simulink model "dynamic_model_euler_copy_to_compare"  (R2021b)
settings: Solver=FixedStepAuto  StartTime=0.0  StopTime=simTime  FixedStep=sim_dt  RelTol=1e-3
undefined symbols (not defined in the file): Angle, Axis, d, g, J_platf, m_mass, m_platf, p, q0, roff, sim_dt, tau, time_1, time_2, u0, umax, w0
libraries: sharedtransform x2, simulink x1, robotcorelib x1, dspindex x1, matrix_library x1
settings Model: Creator=piszy  LastModifiedBy=krzysztof
settings SolverCC: ZeroCrossControl=DisableAll  AlgebraicLoopSolver=TrustRegion
settings DataIOCC: SaveOutput=off  SaveTime=off
settings OptimizationCC: BlockReduction=off  DefaultParameterBehavior=Inlined  BufferReuse=off
settings ModelReferenceCC: ModelReferenceNumInstancesAllowed=Single
settings SFSimCC: CustomCodeUndefinedFunction=UseInterfaceOnly
settings GRTTargetCC: CombineOutputUpdateFcns=off  MatFileLogging=off

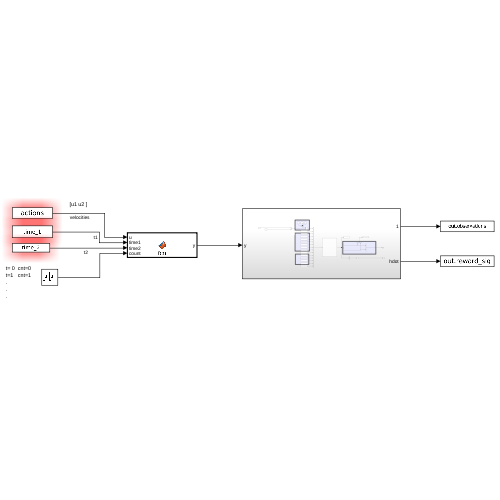
[thumbnail: Simulink's stored preview of the top-level diagram]
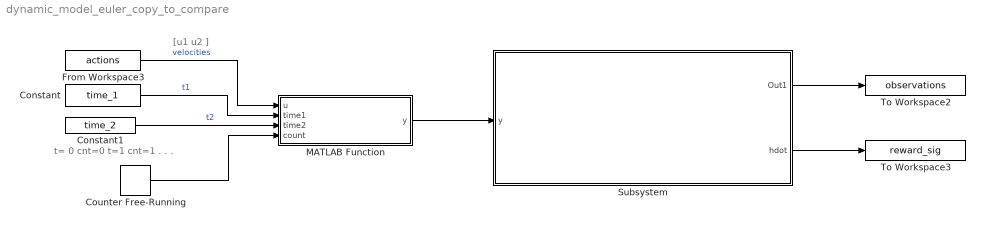
== system dynamic_model_euler_copy_to_compare ==
  note: t= 0  cnt=0
      | t=1   cnt=1
      | .
      | .
      | .
  note: [u1 u2 ]
  Constant : Constant  Value=time_1
  Constant1 : Constant  Value=time_2
  Counter Free-Running : simulink/Sources/Counter Free-Running  NumBits=16  tsamp=-1
  From Workspace3 : FromWorkspace  VariableName=actions
  MATLAB Function : MATLAB Function  TreatAsAtomicUnit=on
  Subsystem : Subsystem
  To Workspace2 : ToWorkspace  VariableName=observations  SampleTime=-1
  To Workspace3 : ToWorkspace  VariableName=reward_sig  SampleTime=-1
  wires:
  Subsystem/1(Out1) -> To Workspace2/1
  Subsystem/2(hdot) -> To Workspace3/1
  From Workspace3/1 -> MATLAB Function/1(u)  "velocities"
  MATLAB Function/1(y) -> Subsystem/1(y)
  Constant/1 -> MATLAB Function/2(time1)  "t1"
  Constant1/1 -> MATLAB Function/3(time2)  "t2"
  Counter Free-Running/1 -> MATLAB Function/4(count)

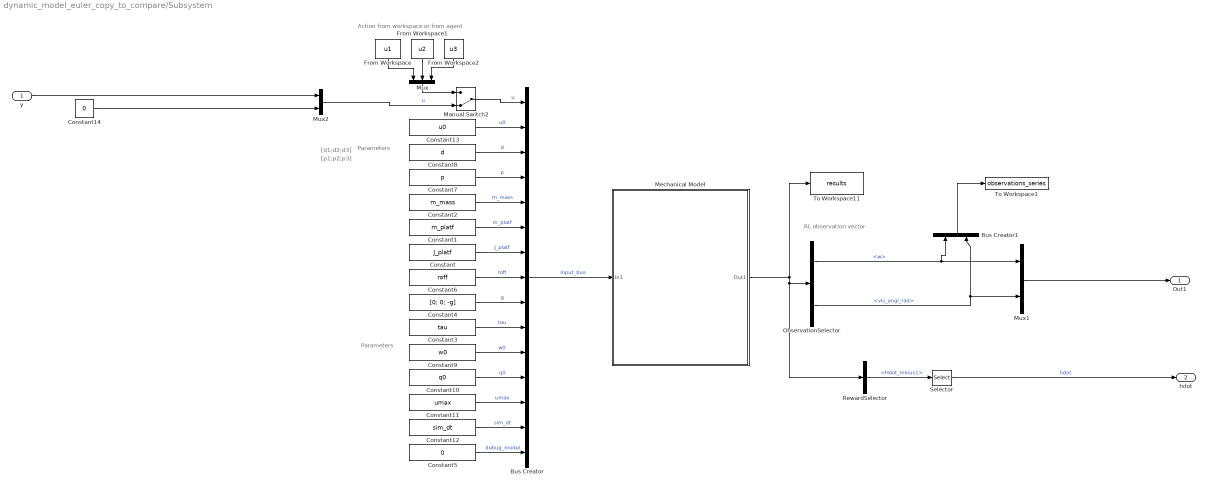
== system dynamic_model_euler_copy_to_compare/Subsystem ==
  note: Parameters
  note: Action from workspace or from agent
  note: RL observation vector
  note: [p1;p2;p3]
  note: [d1;d2;d3]
  note: Parameters
  y : Inport
  Bus Creator : BusCreator  Inputs=15
  Bus Creator1 : BusCreator  Inputs=2
  Constant : Constant  Value=J_platf
  Constant1 : Constant  Value=m_platf
  Constant10 : Constant  Value=q0
  Constant11 : Constant  Value=umax
  Constant12 : Constant  Value=sim_dt
  Constant13 : Constant  Value=u0
  Constant14 : Constant  Value=0
  Constant2 : Constant  Value=m_mass
  Constant3 : Constant  Value=tau
  Constant4 : Constant  Value=[0; 0; -g]
  Constant5 : Constant  Value=0
  Constant6 : Constant  Value=roff
  Constant7 : Constant  Value=p
  Constant8 : Constant  Value=d
  Constant9 : Constant  Value=w0
  From Workspace : FromWorkspace  VariableName=u1
  From Workspace1 : FromWorkspace  VariableName=u2
  From Workspace2 : FromWorkspace  VariableName=u3
  Manual Switch2 : ManualSwitch  CurrentSetting=0
  Mechanical Model : Subsystem
  Mux : Mux  Inputs=3
  Mux1 : Mux  Inputs=2
  Mux2 : Mux  Inputs=2
  ObservationSelector : BusSelector  OutputSignals=w,vis_angl_rad
  RewardSelector : BusSelector  OutputSignals=Hdot_minus1
  Selector : Selector  InputPortWidth=3  IndexOptions=Index vector (dialog)  Indices=[3]  OutputSizes=1
  To Workspace1 : ToWorkspace  VariableName=observations_series  SaveFormat=Timeseries  SampleTime=-1
      settings: Save2DSignal=2-D array (concatenate along first dimension)
  To Workspace11 : ToWorkspace  VariableName=results  SaveFormat=Timeseries  SampleTime=-1
      settings: Save2DSignal=2-D array (concatenate along first dimension)
  Out1 : Outport
  hdot : Outport  Port=2
  wires:
  Constant10/1 -> Bus Creator/12  "q0"
  Constant2/1 -> Bus Creator/5  "m_mass"
  Constant14/1 -> Mux2/2
  Constant11/1 -> Bus Creator/13  "umax"
  Constant13/1 -> Bus Creator/2  "u0"
  Bus Creator1/1 -> To Workspace1/1
  Constant9/1 -> Bus Creator/11  "w0"
  Constant1/1 -> Bus Creator/6  "m_platf"
  Constant7/1 -> Bus Creator/4  "p"
  Constant3/1 -> Bus Creator/10  "tau"
  Constant4/1 -> Bus Creator/9  "g"
  y/1 -> Mux2/1
  Constant6/1 -> Bus Creator/8  "roff"
  ObservationSelector/1 -> Bus Creator1/1, Mux1/1  "<w>"
  Constant12/1 -> Bus Creator/14  "sim_dt"
  Mux1/1 -> Out1/1
  Mechanical Model/1(Out1) -> To Workspace11/1, ObservationSelector/1, RewardSelector/1
  Selector/1 -> hdot/1  "hdot"
  Constant5/1 -> Bus Creator/15  "debug_model"
  Constant/1 -> Bus Creator/7  "J_platf"
  RewardSelector/1 -> Selector/1  "<Hdot_minus1>"
  Constant8/1 -> Bus Creator/3  "d"
  ObservationSelector/2 -> Bus Creator1/2, Mux1/2  "<vis_angl_rad>"
  From Workspace2/1 -> Mux/3
  From Workspace1/1 -> Mux/2
  From Workspace/1 -> Mux/1
  Bus Creator/1 -> Mechanical Model/1(In1)  "input_bus"
  Mux2/1 -> Manual Switch2/2  "u"
  Mux/1 -> Manual Switch2/1
  Manual Switch2/1 -> Bus Creator/1  "u"

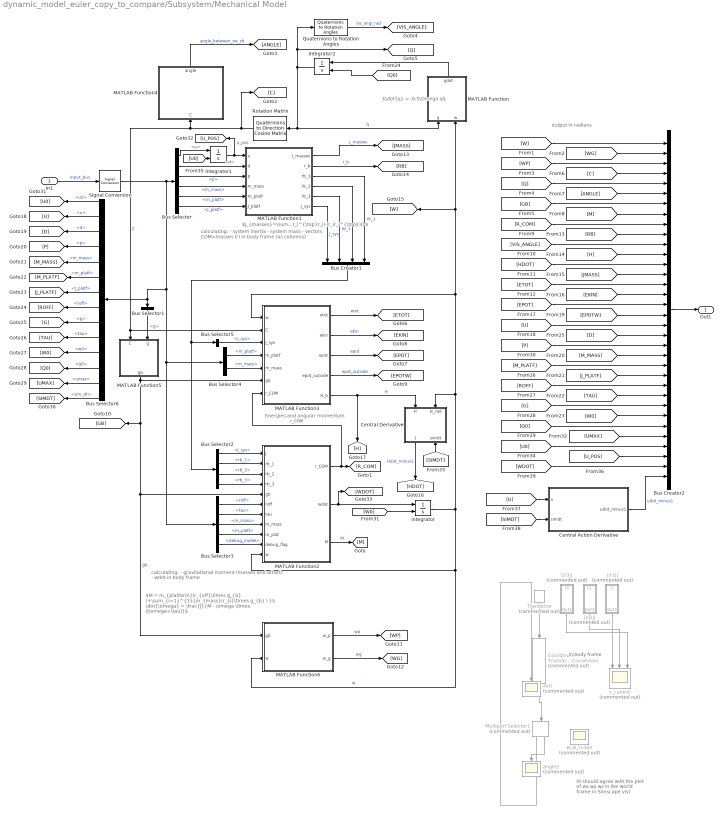
== system dynamic_model_euler_copy_to_compare/Subsystem/Mechanical Model ==
  note: $J_{masses}=\sum_{i=1}^{3}{m_{i}(I(r_i^{\top}r_i)-(r_ir_i^{\top}))}$
  note: $\dot{q} = -0.5\Omega q$
  note: $M = m_{platform}(r_{off}\times g_{b} )+\sum_{i=1}^{3}{m_{mass}(r_{i}\times g_{b} ) }\\ \dot{\omega} = \frac{J}{M - \omega \times (J\omega+\tau)}$
  note: (it should agree with the plot of wx wy wz in the world frame in Simscape vis)
  note: calculating:
      | - system inertia
      | - system mass
      | - vectors COM>masses (r) in body frame
      | (as columns)
  note: calculating:
      | - gravitational moment (masses and offset)
      | - wdot
      | in body frame
  note: in body frame
  note: Energies and angular momentum
  note: output in radians
  In1 : Inport
  Bus Creator1 : BusCreator  Inputs=4
  Bus Creator2 : BusCreator  Inputs=34
  Bus Selector : BusSelector  OutputSignals=u,d,p,m_mass,m_platf,J_platf
  Bus Selector1 : BusSelector  OutputSignals=g
  Bus Selector2 : BusSelector  OutputSignals=J_sys,rb_1,rb_2,rb_3
  Bus Selector3 : BusSelector  OutputSignals=roff,tau,m_mass,m_platf,debug_model
  Bus Selector4 : BusSelector  OutputSignals=m_platf,m_mass
  Bus Selector5 : BusSelector  OutputSignals=J_sys
  Bus Selector6 : BusSelector  OutputSignals=u0,u,d,p,m_mass,m_platf,J_platf,roff,g,tau,w0,q0,umax,sim_dt
  Central Action Derivative : Subsystem
  Central Derivative : Subsystem
      settings: PortSchema="{\"entries\":[{\"content\":{\"sides\":[{\"content\":{\"connectorIds\":[\"In1\",\"In2\"]},\"type\":\"ConnectorPlacement.EquallySpacedRectSide\",\"uuid\":\"1383cf58-ed2e-4d76-b2bd-bc812874c5c5\"},{\"content\":{\"connectorIds\":[\"Out1\",\"In3\"],\"side\":\"RIGHT\"},\"type\":\"ConnectorPlacement.EquallySpacedRectSide\",\"uuid\":\"b1333be6-c310-4c35-a541-4e98fbac6c75\"},{\"content\":{\"connectorIds\":[],\"side\":\"TOP\"},\"type\":\"ConnectorPlacement.EquallySpacedRectSide\",\"uuid\":\"9de10ece-9fa2-48e9-be23-db895089292f\"}]},\"type\":\"ConnectorPlacement.EquallySpacedConnector\",\"uuid\":\"8dd4b87f-23e7-464d-a0c4-c49a8f880c8a\"}],\"packageUris\":[\"http://schema.mathworks.com/mf0/Connector/R2020b\"],\"version\":\"1.0\"}"
  Coordinate Transformation Conversion : robotcorelib/Coordinate Transformation Conversion  Commented=on  InputRepresentation=Rotation Matrix  InputEulerSequence=ZYX  ShowTrVecInputPort=on  OutputRepresentation=Axis-Angle  OutputEulerSequence=ZYX  ShowTrVecOutputPort=on  SimulateUsing=Interpreted execution
      settings: SourceProductBaseCode=NV,RO,RR,UV
  Integrator : Integrator  InitialConditionSource=external
  Integrator1 : Integrator  InitialConditionSource=external
  Integrator2 : Integrator  InitialConditionSource=external
  MATLAB Function : MATLAB Function  TreatAsAtomicUnit=on
  MATLAB Function1 : MATLAB Function  TreatAsAtomicUnit=on
  MATLAB Function2 : MATLAB Function  TreatAsAtomicUnit=on
  MATLAB Function3 : MATLAB Function  TreatAsAtomicUnit=on
  MATLAB Function4 : MATLAB Function  TreatAsAtomicUnit=on
  MATLAB Function5 : MATLAB Function  TreatAsAtomicUnit=on
  MATLAB Function6 : MATLAB Function  TreatAsAtomicUnit=on
  Multiport Selector1 : dspindex/Multiport Selector  Commented=on  rowsOrCols=Rows  idxCellArray={1:3,4}  idxErrMode=Clip Index
  Quaternions to Rotation Angles : sharedtransform/Quaternions to Rotation Angles  rotationOrder=XYZ  aMode=aMode
      settings: SourceProductBaseCode=AE,PW,DR,MT,UV,VE
  Rotation Matrix : sharedtransform/Quaternions to  Direction Cosine Matrix  aMode=aMode
      settings: SourceProductBaseCode=AE,PW,DR,MT,UV,VE
  Signal Conversion : SignalConversion  OverrideOpt=on
  Transpose : matrix_library/Transpose  Commented=on
      settings: SourceProductBaseCode=SL
  angle2 : Scope  Commented=on
  axis : Scope  Commented=on
  r_control : Scope  Commented=on  NumInputPorts=3
  w_w_scope : Scope  Commented=on
  ||r1|| : Subsystem  Commented=on
  ||r2|| : Subsystem  Commented=on
  ||r3|| : Subsystem  Commented=on
  Out1 : Outport
  wires:
  Integrator2/1 -> MATLAB Function/1(q), Rotation Matrix/1, [Q], Quaternions to Rotation Angles/1  "q"
  MATLAB Function/1(qdot) -> Integrator2/1
  Transpose/1 -> Coordinate Transformation Conversion/1
  Coordinate Transformation Conversion/1 -> Multiport Selector1/1
  Multiport Selector1/2 -> angle2/1
  Multiport Selector1/1 -> axis/1
  ||r3||/1(Out1) -> r_control/3
  ||r1||/1(Out1) -> r_control/1
  ||r2||/1(Out1) -> r_control/2
  In1/1 -> Signal Conversion/1  "input_bus"
  Bus Selector/2 -> MATLAB Function1/2(d)  "<d>"
  Bus Selector/3 -> MATLAB Function1/3(p)  "<p>"
  Bus Selector/4 -> MATLAB Function1/4(m_mass)  "<m_mass>"
  Bus Selector/5 -> MATLAB Function1/5(m_platf)  "<m_platf>"
  Bus Selector1/1 -> MATLAB Function5/2(g)  "<g>"
  MATLAB Function2/2(wdot) -> Integrator/1, [WDOT]
  Integrator/1 -> MATLAB Function6/2(w), MATLAB Function2/11(w), MATLAB Function3/1(w), [W], MATLAB Function/2(w), Central Derivative/2(w_rad)  "w"
  MATLAB Function1/3(rb_1) -> Bus Creator1/4  "rb_1"
  MATLAB Function5/1(gb) -> MATLAB Function6/1(gb), MATLAB Function2/5(gb), [GB], MATLAB Function3/6(gb)  "gb"
  MATLAB Function1/4(rb_2) -> Bus Creator1/3  "rb_2"
  MATLAB Function1/5(rb_3) -> Bus Creator1/2  "rb_3"
  MATLAB Function1/6(J_sys) -> Bus Creator1/1  "J_sys"
  Bus Selector3/1 -> MATLAB Function2/6(roff)  "<roff>"
  Bus Selector3/2 -> MATLAB Function2/7(tau)  "<tau>"
  Bus Selector3/3 -> MATLAB Function2/8(m_mass)  "<m_mass>"
  Bus Selector3/4 -> MATLAB Function2/9(m_plat)  "<m_platf>"
  Bus Creator1/1 -> Bus Selector5/1, Bus Selector2/1
  MATLAB Function2/3(M) -> [M]  "M"
  MATLAB Function3/2(ekin) -> [EKIN]  "ekin"
  MATLAB Function3/3(epot) -> [EPOT]  "epot"
  MATLAB Function3/1(etot) -> [ETOT]  "etot"
  MATLAB Function6/1(w_p) -> [WP]  "wp"
  MATLAB Function6/2(w_g) -> [WG]  "wg"
  MATLAB Function1/1(J_masses) -> [JMASS]  "J_masses"
  Bus Selector/6 -> MATLAB Function1/6(J_platf)  "<J_platf>"
  Bus Selector3/5 -> MATLAB Function2/10(debug_flag)  "<debug_model>"
  Bus Selector4/2 -> MATLAB Function3/5(m_mass)  "<m_mass>"
  Bus Selector4/1 -> MATLAB Function3/4(m_platf)  "<m_platf>"
  MATLAB Function2/1(r_COM) -> [R_COM], MATLAB Function3/7(r_COM)  "r_COM"
  Bus Selector2/1 -> MATLAB Function2/1(J)  "<J_sys>"
  Bus Selector2/3 -> MATLAB Function2/3(rb_2)  "<rb_2>"
  Bus Selector2/2 -> MATLAB Function2/2(rb_1)  "<rb_1>"
  Bus Selector2/4 -> MATLAB Function2/4(rb_3)  "<rb_3>"
  Bus Selector5/1 -> MATLAB Function3/3(J_sys)  "<J_sys>"
  MATLAB Function3/4(epot_outside) -> [EPOTW]  "epot_outside"
  Rotation Matrix/1 -> [C], MATLAB Function3/2(C), MATLAB Function5/1(C), MATLAB Function4/1(C)  "C"
  Bus Creator2/1 -> Out1/1
  MATLAB Function1/2(r_b) -> [RB]  "r_b"
  MATLAB Function4/1(angle) -> [ANGLE]  "angle_between_zw_zb"
  Quaternions to Rotation Angles/1 -> [VIS_ANGLE]  "vis_angl_rad"
  [W] -> Bus Creator2/1
  [WG] -> Bus Creator2/2
  [C] -> Bus Creator2/4
  [WP] -> Bus Creator2/3
  [JMASS] -> Bus Creator2/14
  [HDOT] -> Bus Creator2/13
  [H] -> Bus Creator2/12
  [VIS_ANGLE] -> Bus Creator2/11
  [R_COM] -> Bus Creator2/9
  [ETOT] -> Bus Creator2/15
  [EPOT] -> Bus Creator2/17
  [EPOTW] -> Bus Creator2/18
  [Q] -> Bus Creator2/5
  [GB] -> Bus Creator2/7
  [ANGLE] -> Bus Creator2/6
  [M] -> Bus Creator2/8
  [RB] -> Bus Creator2/10
  [EKIN] -> Bus Creator2/16
  [U] -> Bus Creator2/19
  Bus Selector6/7 -> [J_PLATF]  "<J_platf>"
  Bus Selector6/8 -> [ROFF]  "<roff>"
  Bus Selector6/9 -> [G]  "<g>"
  Bus Selector6/10 -> [TAU]  "<tau>"
  Bus Selector6/11 -> [W0]  "<w0>"
  Bus Selector6/12 -> [Q0]  "<q0>"
  Bus Selector6/6 -> [M_PLATF]  "<m_platf>"
  Bus Selector6/5 -> [M_MASS]  "<m_mass>"
  Bus Selector6/4 -> [P]  "<p>"
  Bus Selector6/3 -> [D]  "<d>"
  Bus Selector6/2 -> [U]  "<u>"
  [D] -> Bus Creator2/20
  [TAU] -> Bus Creator2/26
  [M_MASS] -> Bus Creator2/22
  [W0] -> Bus Creator2/28
  [J_PLATF] -> Bus Creator2/24
  [P] -> Bus Creator2/21
  [M_PLATF] -> Bus Creator2/23
  [ROFF] -> Bus Creator2/25
  [G] -> Bus Creator2/27
  [Q0] -> Bus Creator2/29
  [Q0] -> Integrator2/2
  [W0] -> Integrator/2
  MATLAB Function3/5(H_b) -> Central Derivative/1(H), [H]  "H"
  Central Derivative/1(Hdot_minus1) -> [HDOT]  "Hdot_minus1"
  Bus Selector6/13 -> [UMAX]  "<umax>"
  [UMAX] -> Bus Creator2/30
  Bus Selector6/14 -> [SIMDT]  "<sim_dt>"
  [SIMDT] -> Central Derivative/3(simdt)
  Signal Conversion/1 -> Bus Selector3/1, Bus Selector4/1, Bus Selector1/1, Bus Selector6/1, Bus Selector/1
  Bus Selector6/1 -> [U0]  "<u0>"
  [U0] -> Bus Creator2/31
  Bus Selector/1 -> Integrator1/1  "<u>"
  [U0] -> Integrator1/2
  Integrator1/1 -> [U_POS], MATLAB Function1/1(u)  "u_pos"
  [U_POS] -> Bus Creator2/32
  [U] -> Central Action Derivative/2(u)
  [SIMDT] -> Central Action Derivative/1(simdt)
  Central Action Derivative/1(udot_minus1) -> Bus Creator2/34  "udot_minus1"
  [WDOT] -> Bus Creator2/33

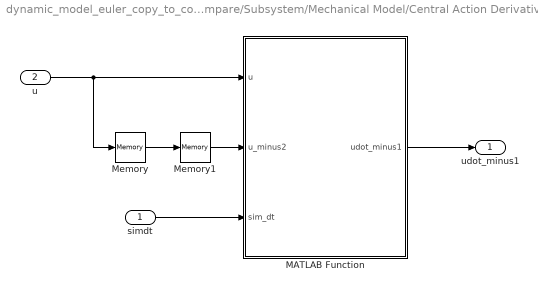
== system dynamic_model_euler_copy_to_compare/Subsystem/Mechanical Model/Central Action Derivative ==
  simdt : Inport
  u : Inport  Port=2
  MATLAB Function : MATLAB Function  TreatAsAtomicUnit=on
  Memory : Memory
  Memory1 : Memory
  udot_minus1 : Outport
  wires:
  u/1 -> Memory/1, MATLAB Function/1(u)
  simdt/1 -> MATLAB Function/3(sim_dt)
  Memory/1 -> Memory1/1
  MATLAB Function/1(udot_minus1) -> udot_minus1/1
  Memory1/1 -> MATLAB Function/2(u_minus2)

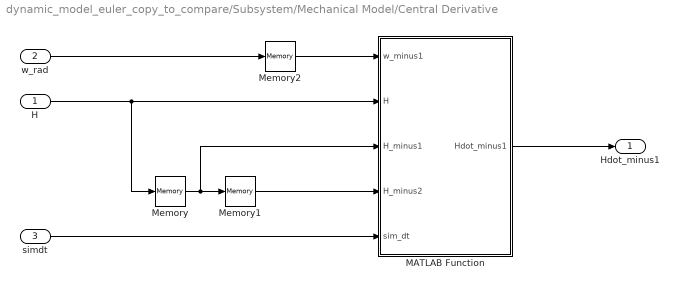
== system dynamic_model_euler_copy_to_compare/Subsystem/Mechanical Model/Central Derivative ==
  H : Inport
  w_rad : Inport  Port=2
  simdt : Inport  Port=3
  MATLAB Function : MATLAB Function  TreatAsAtomicUnit=on
  Memory : Memory
  Memory1 : Memory
  Memory2 : Memory
  Hdot_minus1 : Outport
  wires:
  Memory1/1 -> MATLAB Function/4(H_minus2)
  H/1 -> MATLAB Function/2(H), Memory/1
  Memory2/1 -> MATLAB Function/1(w_minus1)
  simdt/1 -> MATLAB Function/5(sim_dt)
  Memory/1 -> MATLAB Function/3(H_minus1), Memory1/1
  MATLAB Function/1(Hdot_minus1) -> Hdot_minus1/1
  w_rad/1 -> Memory2/1

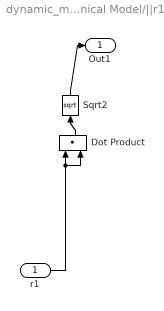
== system dynamic_model_euler_copy_to_compare/Subsystem/Mechanical Model/||r1|| ==
  r1 : Inport
  Dot Product : DotProduct  RndMeth=Nearest  InputSameDT=on  OutDataTypeStr=Inherit: Inherit via internal rule
  Sqrt2 : Sqrt  SaturateOnIntegerOverflow=on
  Out1 : Outport
  wires:
  Dot Product/1 -> Sqrt2/1
  r1/1 -> Dot Product/2, Dot Product/1
  Sqrt2/1 -> Out1/1

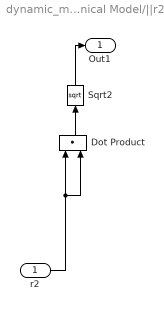
== system dynamic_model_euler_copy_to_compare/Subsystem/Mechanical Model/||r2|| ==
  r2 : Inport
  Dot Product : DotProduct  RndMeth=Nearest  InputSameDT=on  OutDataTypeStr=Inherit: Inherit via internal rule
  Sqrt2 : Sqrt  SaturateOnIntegerOverflow=on
  Out1 : Outport
  wires:
  Dot Product/1 -> Sqrt2/1
  r2/1 -> Dot Product/1, Dot Product/2
  Sqrt2/1 -> Out1/1

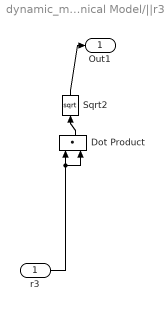
== system dynamic_model_euler_copy_to_compare/Subsystem/Mechanical Model/||r3|| ==
  r3 : Inport
  Dot Product : DotProduct  RndMeth=Nearest  InputSameDT=on  OutDataTypeStr=Inherit: Inherit via internal rule
  Sqrt2 : Sqrt  SaturateOnIntegerOverflow=on
  Out1 : Outport
  wires:
  Dot Product/1 -> Sqrt2/1
  r3/1 -> Dot Product/2, Dot Product/1
  Sqrt2/1 -> Out1/1

== matlab function dynamic_model_euler_copy_to_compare/Subsystem/Mechanical Model/Central Derivative/MATLAB Function ==
  data: w_minus1 input; H input; H_minus1 input; Hdot_minus1 output; H_minus2 input; sim_dt input
function Hdot_minus1 = fcn(w_minus1,H,H_minus1,H_minus2, sim_dt)
   H_in_body_dot_minus1 = (H - H_minus2)/2/sim_dt;
   Hdot_minus1 = H_in_body_dot_minus1 + cross(w_minus1,H_minus1);

== matlab function dynamic_model_euler_copy_to_compare/Subsystem/Mechanical Model/Central Action Derivative/MATLAB Function ==
  data: u input; u_minus2 input; udot_minus1 output; sim_dt input
function udot_minus1 = fcn(u,u_minus2, sim_dt)
   udot_minus1 = (u - u_minus2)/2/sim_dt;

== matlab function dynamic_model_euler_copy_to_compare/MATLAB Function ==
  data: u input; y output; time1 input; time2 input; count input
function y = fcn(u,time1, time2, count)
    action1 = u(1); action2 = u(2);
    y = zeros(2,1);

    if count<=time1, y(1) = action1;
    else, y(1) = 0;end

    if count<=time2, y(2) = action2;
    else, y(2) = 0;end

== matlab function dynamic_model_euler_copy_to_compare/Subsystem/Mechanical Model/MATLAB Function5 ==
  data: C input; gb output; g input
function gb = gbodyframe(C,g)
gb = C*g;

== matlab function dynamic_model_euler_copy_to_compare/Subsystem/Mechanical Model/MATLAB Function3 ==
  data: w input; C input; J_sys input; m_platf input; m_mass input; gb input; etot output; ekin output; epot output; epot_outside output; H_b output; r_COM input
function [etot,ekin,epot,epot_outside, H_b] = fcn(w,C,J_sys, m_platf,m_mass,gb,r_COM)
% J_sys = concat_in(:,1:3);
% rb1 = concat_in(:,6);
% rb2 = concat_in(:,5);
% rb3 = concat_in(:,4);

% disp(r_COM)

ekin = 0.5*(w)'*J_sys*(w);

epot = (3*m_mass + m_platf) * gb(3) * vecnorm(r_COM);
%epot = m_platf*gb(3)*vecnorm(r_COM);

r_COM_w = C'*r_COM;
epot_outside = (3*m_mass + m_platf) * vecnorm(gb) * r_COM_w(3);

etot = epot+ekin;
%hmag = vecnorm(J*w);

% H_b = [J_sys(1,1)*w(1)-J_sys(1,2)*w(2)-J_sys(1,3)*w(3); 
%     -J_sys(2,1)*w(1)+J_sys(2,2)*w(2)-J_sys(2,3)*w(3); 
%     -J_sys(3,1)*w(1)-J_sys(3,2)*w(2)+J_sys(3,3)*w(3); 
%     ];

H_b = J_sys * w;

== matlab function dynamic_model_euler_copy_to_compare/Subsystem/Mechanical Model/MATLAB Function ==
  data: q input; w input; qdot output
function qdot = derq(q,w)

w_x = w(1); w_y = w(2); w_z = w(3);

% omega = [ 0     w_z   -w_y    w_x;... 
%           -w_z   0       w_x    w_y;... 
%           w_y   -w_x    0       w_z;... 
%           -w_x   -w_y    -w_z     0];

omega = [ 0      w_x   w_y    w_z;... 
          -w_x   0    -w_z    w_y;... 
          -w_y   w_z    0    -w_x;... 
          -w_z  -w_y   w_x     0];

qdot = -0.5*omega*q;

== matlab function dynamic_model_euler_copy_to_compare/Subsystem/Mechanical Model/MATLAB Function2 ==
  data: r_COM output; J input; rb_1 input; rb_2 input; rb_3 input; gb input; roff input; tau input; m_mass input; m_plat input; debug_flag input; w input; wdot output; M output
function [r_COM, wdot, M] = fcn(J, rb_1, rb_2, rb_3, gb, roff, tau, m_mass, m_plat, debug_flag,w)

% concatenated along columns
% J = concat_in(:,1:3);
% rb_1 = concat_in(:,6);
% rb_2 = concat_in(:,5);
% rb_3 = concat_in(:,4);
if debug_flag
    disp("Inside gravitational torque and wdot calculation function:")
    disp("J"),disp(J)
    disp("rb1"),disp(rb_1)
    disp("rb2"),disp(rb_2)
    disp("rb3"),disp(rb_3)
    disp("gb"),disp(gb)
    disp("roff"),disp(roff)
    disp("tau"),disp(tau)
    disp("w"),disp(w)
end

r_COM = (m_mass*rb_1 + m_mass*rb_2 + m_mass*rb_3 + m_plat*roff)/(3*m_mass+m_plat);

%M = m_plat*cross(roff,gb) + m_mass*cross(rb_1,gb) + m_mass*cross(rb_2,gb) + m_mass*cross(rb_3,gb);
M = (3*m_mass+m_plat)*cross(r_COM,gb);

wdot = J\(M-cross(w,(J*w))+tau); %given that dt(Jw)/dt = J * dw/dt

== matlab function dynamic_model_euler_copy_to_compare/Subsystem/Mechanical Model/MATLAB Function1 ==
  data: J_masses output; r_b output; rb_1 output; rb_2 output; rb_3 output; J_sys output; u input; d input; p input; m_mass input; m_platf input; J_platf input
function [J_masses, r_b, rb_1, rb_2, rb_3,  J_sys] = fcn(u, d, p, m_mass, m_platf, J_platf)
% [r1x r1y r1z; r2x r2y r2z; r3x r3y r3z]
% [p1x p1y p1z; p2x p2y p2z; p3x p3y p3z]
% [	d1x d1y d1z; 
% 	d2x d2y d2z; 
% 	d3x d3y d3z]
% [u1; u2; u3] !!!!==== jestem przekonany, że to kolumna
% r = p + u/||d||*d
% r is a sum of the p vector and a vector of length u that is along
% d vector

% d' = 	[d1x d2x d3x; 
%		 d1y d2y d3y; 
%		 d1z d2z d3z]
% vecnorm(d') = 	[||d1|| ||d2|| ||d3||]
% (vecnorm(d'))' = 	[||d1||;||d2||;||d3||]
% (u ./ (vecnorm(d'))') = [u1/||d1||; u2/||d2||; u3/||d3||]
% (u ./ (vecnorm(d'))') .* d = [	u1/||d1||*d1x	u1/||d1||*d1y u1/||d1||*d1z;
%								    u2/||d2||*d2x	u2/||d2||*d2y u2/||d2||*d2z;
%								    u3/||d3||*d3x	u3/||d3||*d3y u3/||d3||*d3z;
r_b = p + (u ./ (vecnorm(d'))') .* d;

% make rb column vectors
rb_1 = r_b(1,:)'; rb_2 = r_b(2,:)'; rb_3 = r_b(3,:)'; 

J_masses =    m_mass*(eye(3)*(rb_1' * rb_1) - rb_1 * rb_1')...
            + m_mass*(eye(3)*(rb_2' * rb_2) - rb_2 * rb_2')... 
            + m_mass*(eye(3)*(rb_3' * rb_3) - rb_3 * rb_3');

% to Eq. 6 in (Zagórski 2020)

J_sys = J_masses + J_platf;
% m_sys = m_platf + 3 * m_mass;

== matlab function dynamic_model_euler_copy_to_compare/Subsystem/Mechanical Model/MATLAB Function4 ==
  data: C input; angle output
function angle    = calculate_constraint(C)
%     rw1 = Q'*r1;
%     rw2 = Q'*r2;
%     rw3 = Q'*r3;
%     w_w = Q'*w;
    % k_prim - coordinates of body frame versor in the inertial frame
    k_prim = C' * [0; 0; 1];
    % angle = acos( round( dot( k_prim, [0; 0; 1]) * 1e13) / 1e13); 
    angle = acos ( round( k_prim(3) * 1e13 ) / 1e13);
    % beacuse [0; 0; 1] => k_prim_x*0 and k_prim_y*0
    % and ||k||||k'|| = 1
    % rounding to 13 decimal places to get rid of the situation that cos due to calculation error > 1
end

== matlab function dynamic_model_euler_copy_to_compare/Subsystem/Mechanical Model/MATLAB Function6 ==
  data: gb input; w input; w_p output; w_g output
function [w_p, w_g] = projection_operator(gb,w)
operator =  eye - (gb * gb')/((vecnorm(gb))^2);
w_p = (operator * w);
w_g = (w - w_p);
